simulink model "Impedance"  (R2020a)
settings: Solver=VariableStepAuto  StartTime=0.0  StopTime=2.0  RelTol=1e-3
values from neighbouring files (symbols this model uses):
  g = 9.81    [params.m]
  KD = 2*z*w    [params.m]
  KP = w^2    [params.m]
  Md = diag([2 2 2 2 2 2])    [params.m]
libraries: vrlib x1
settings Model: Creator=Sebastiano  LastModifiedBy=Sebastiano

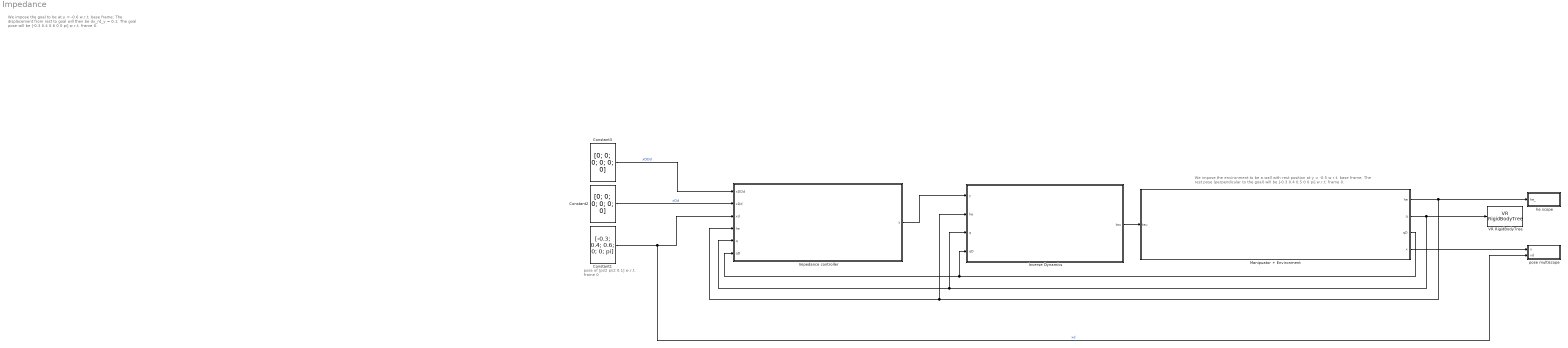
== system Impedance ==
  note: pose of [pi/2 pi/2 0.1]
      | w.r.t. frame 0
  note: We impose the environment to be a wall with rest position at y = -0.5 w.r.t. base frame;
      | The rest pose (perpendicular to the goal) will be [-0.3 0.4 0.5 0 0 pi] w.r.t. frame 0.
  note: We impose the goal to be at y = -0.6 w.r.t. base frame;
      | The displacement from rest to goal will then be dx_rd_y = 0.1;
      | The goal pose will be [-0.3 0.4 0.6 0 0 pi] w.r.t. frame 0.
  Constant1 : Constant  Value=[-0.3; 0.4; 0.6; 0; 0; pi]  VectorParams1D=off
  Constant2 : Constant  Value=[0; 0; 0; 0; 0; 0]  VectorParams1D=off
  Constant3 : Constant  Value=[0; 0; 0; 0; 0; 0]  VectorParams1D=off
  Impedance controller : Subsystem
  Inverse Dynamics : Subsystem
  Manipuator + Environment : Subsystem
  VR RigidBodyTree : vrlib/VR RigidBodyTree  RBT=robot  useRBT=on  Ts=-1  ForceViewerOpen=on
      settings: SourceProductBaseCode=SL
  he scope : Subsystem
  pose multiscope : Subsystem
  wires:
  Constant1/1 -> pose multiscope/2(xd), Impedance controller/3(xd)  "xd"
  Constant3/1 -> Impedance controller/1(xDDd)  "xDDd"
  Constant2/1 -> Impedance controller/2(xDd)  "xDd"
  Impedance controller/1(y) -> Inverse Dynamics/1(y)
  Manipuator + Environment/3(qD) -> Inverse Dynamics/4(qD), Impedance controller/6(qD)
  Manipuator + Environment/2(q) -> VR RigidBodyTree/1, Inverse Dynamics/3(q), Impedance controller/5(q)
  Inverse Dynamics/1(tau) -> Manipuator + Environment/1(tau)
  Manipuator + Environment/1(he) -> he scope/1(he_), Impedance controller/4(he), Inverse Dynamics/2(he)
  Manipuator + Environment/4(x) -> pose multiscope/1(x)

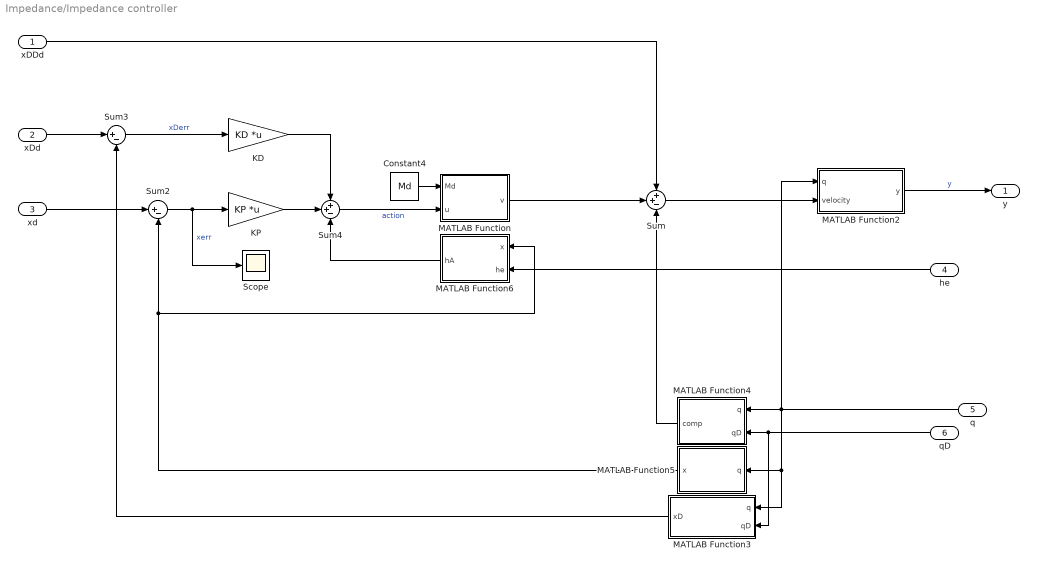
== system Impedance/Impedance controller ==
  xDDd : Inport
  xDd : Inport  Port=2
  xd : Inport  Port=3
  he : Inport  Port=4
  q : Inport  Port=5
  qD : Inport  Port=6
  Constant4 : Constant  Value=Md
  KD : Gain  Gain=KD  Multiplication=Matrix(K*u) (u vector)
  KP : Gain  Gain=KP  Multiplication=Matrix(K*u) (u vector)
  MATLAB Function : MATLAB Function  TreatAsAtomicUnit=on
  MATLAB Function2 : MATLAB Function  TreatAsAtomicUnit=on
  MATLAB Function3 : MATLAB Function  TreatAsAtomicUnit=on
  MATLAB Function4 : MATLAB Function  TreatAsAtomicUnit=on
  MATLAB Function5 : MATLAB Function  TreatAsAtomicUnit=on
  MATLAB Function6 : MATLAB Function  TreatAsAtomicUnit=on
  Scope : Scope
  Sum : Sum  Inputs=++-
  Sum2 : Sum  Inputs=|+-
  Sum3 : Sum  Inputs=|+-
  Sum4 : Sum  Inputs=++-
  y : Outport
  wires:
  Sum/1 -> MATLAB Function2/2(velocity)
  q/1 -> MATLAB Function3/1(q), MATLAB Function5/1(q), MATLAB Function4/1(q), MATLAB Function2/1(q)
  MATLAB Function5/1(x) -> Sum2/2, MATLAB Function6/1(x)
  xd/1 -> Sum2/1
  xDd/1 -> Sum3/1
  he/1 -> MATLAB Function6/2(he)
  Constant4/1 -> MATLAB Function/1(Md)
  MATLAB Function2/1(y) -> y/1  "y"
  qD/1 -> MATLAB Function4/2(qD), MATLAB Function3/2(qD)
  MATLAB Function3/1(xD) -> Sum3/2
  MATLAB Function4/1(comp) -> Sum/3
  Sum3/1 -> KD/1  "xDerr"
  xDDd/1 -> Sum/1
  KD/1 -> Sum4/1
  Sum2/1 -> Scope/1, KP/1  "xerr"
  KP/1 -> Sum4/2
  MATLAB Function/1(v) -> Sum/2
  Sum4/1 -> MATLAB Function/2(u)  "action"
  MATLAB Function6/1(hA) -> Sum4/3

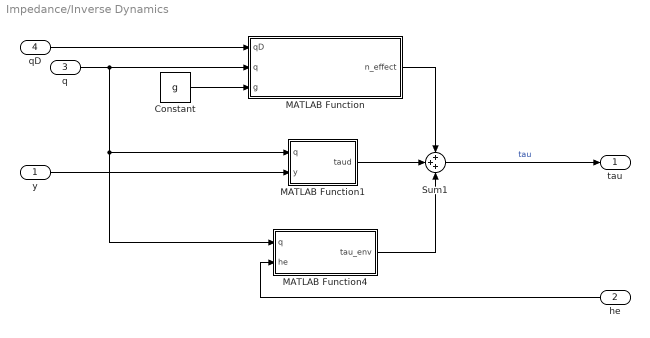
== system Impedance/Inverse Dynamics ==
  y : Inport
  he : Inport  Port=2
  q : Inport  Port=3
  qD : Inport  Port=4
  Constant : Constant  Value=g
  MATLAB Function : MATLAB Function  TreatAsAtomicUnit=on
  MATLAB Function1 : MATLAB Function  TreatAsAtomicUnit=on
  MATLAB Function4 : MATLAB Function  TreatAsAtomicUnit=on
  Sum1 : Sum  Inputs=+++
  tau : Outport
  wires:
  qD/1 -> MATLAB Function/1(qD)
  MATLAB Function/1(n_effect) -> Sum1/1
  MATLAB Function1/1(taud) -> Sum1/2
  q/1 -> MATLAB Function/2(q), MATLAB Function4/1(q), MATLAB Function1/1(q)
  Constant/1 -> MATLAB Function/3(g)
  y/1 -> MATLAB Function1/2(y)
  Sum1/1 -> tau/1  "tau"
  MATLAB Function4/1(tau_env) -> Sum1/3
  he/1 -> MATLAB Function4/2(he)

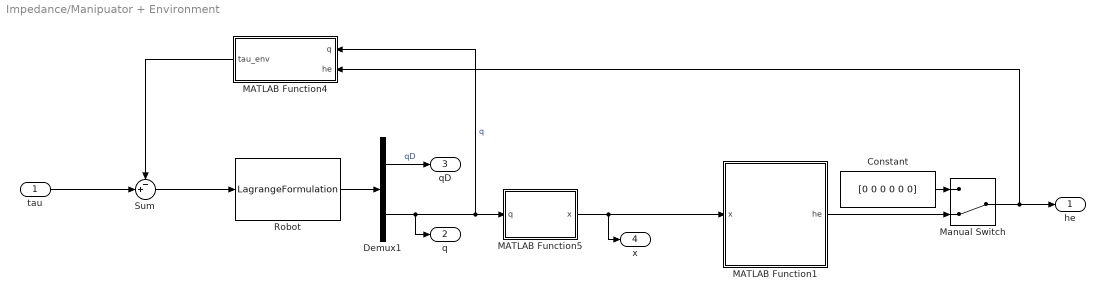
== system Impedance/Manipuator + Environment ==
  tau : Inport
  Constant : Constant  Value=[0 0 0 0 0 0]
  Demux1 : Demux  Outputs=[3, 3]
  MATLAB Function1 : MATLAB Function  TreatAsAtomicUnit=on
  MATLAB Function4 : MATLAB Function  TreatAsAtomicUnit=on
  MATLAB Function5 : MATLAB Function  TreatAsAtomicUnit=on
  Manual Switch : ManualSwitch  CurrentSetting=0
  Robot : S-Function  FunctionName=LagrangeFormulation  Parameters=g  SFunctionDeploymentMode=off  EnableBusSupport=off
  Sum : Sum  Inputs=-+|
  he : Outport
  q : Outport  Port=2
  qD : Outport  Port=3
  x : Outport  Port=4
  wires:
  Sum/1 -> Robot/1
  MATLAB Function1/1(he) -> Manual Switch/2
  Robot/1 -> Demux1/1
  MATLAB Function4/1(tau_env) -> Sum/1
  MATLAB Function5/1(x) -> x/1, MATLAB Function1/1(x)
  Constant/1 -> Manual Switch/1
  Manual Switch/1 -> MATLAB Function4/2(he), he/1
  Demux1/2 -> MATLAB Function4/1(q), MATLAB Function5/1(q), q/1  "q"
  tau/1 -> Sum/2
  Demux1/1 -> qD/1  "qD"

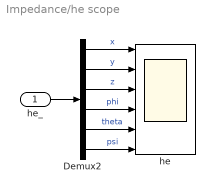
== system Impedance/he scope ==
  he_ : Inport
  Demux2 : Demux  Outputs=[1, 1, 1, 1, 1, 1]
  he : Scope  NumInputPorts=6
  wires:
  Demux2/4 -> he/4  "phi"
  Demux2/3 -> he/3  "z"
  Demux2/6 -> he/6  "psi"
  Demux2/5 -> he/5  "theta"
  Demux2/1 -> he/1  "x"
  he_/1 -> Demux2/1
  Demux2/2 -> he/2  "y"

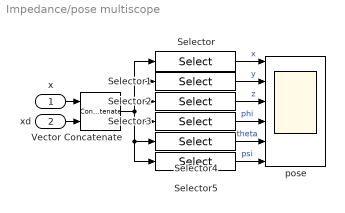
== system Impedance/pose multiscope ==
  x : Inport
  xd : Inport  Port=2
  Selector : Selector  NumberOfDimensions=2  InputPortWidth=3  IndexOptions=Index vector (dialog),Select all  Indices=1,7  OutputSizes=6,6
  Selector1 : Selector  NumberOfDimensions=2  InputPortWidth=3  IndexOptions=Index vector (dialog),Select all  Indices=2,7  OutputSizes=6,6
  Selector2 : Selector  NumberOfDimensions=2  InputPortWidth=3  IndexOptions=Index vector (dialog),Select all  Indices=3,7  OutputSizes=6,6
  Selector3 : Selector  NumberOfDimensions=2  InputPortWidth=3  IndexOptions=Index vector (dialog),Select all  Indices=4,7  OutputSizes=6,6
  Selector4 : Selector  NumberOfDimensions=2  InputPortWidth=3  IndexOptions=Index vector (dialog),Select all  Indices=5,7  OutputSizes=6,6
  Selector5 : Selector  NumberOfDimensions=2  InputPortWidth=3  IndexOptions=Index vector (dialog),Select all  Indices=6,7  OutputSizes=6,6
  Vector Concatenate : Concatenate  Mode=Multidimensional array  ConcatenateDimension=2
  pose : Scope  NumInputPorts=6
  wires:
  x/1 -> Vector Concatenate/1
  xd/1 -> Vector Concatenate/2
  Selector1/1 -> pose/2  "y"
  Selector5/1 -> pose/6  "psi"
  Selector3/1 -> pose/4  "phi"
  Selector/1 -> pose/1  "x"
  Selector4/1 -> pose/5  "theta"
  Vector Concatenate/1 -> Selector/1, Selector1/1, Selector2/1, Selector5/1, Selector4/1, Selector3/1
  Selector2/1 -> pose/3  "z"

== matlab function Impedance/Manipuator + Environment/MATLAB Function1 ==
  data: x input; he output
function he = environment(x)

% environment params
K = diag([2 2 2 0.1 0.1 0.1]);    % stiffness
wall = 0.5; % constraint position w.r.t. frame 0 (it's y=-0.5 w.r.t. base frame)

if x(3) >= wall  % check is done in frame 0
    % touching the environment! constrained motion
    % set up the rest position frame
    % (basically, same orientation as ee but position is the contact point at the wall)
    xr = x;
    xr(3) = wall;
    % calculate the forces
    dx_re = x - xr;
    he = K * dx_re;
else
    % free motion
    he = zeros(6,1);
end

he = reshape(he,[6 1]);

== matlab function Impedance/Manipuator + Environment/MATLAB Function4 ==
  data: q input; he input; tau_env output
function tau_env = J(q, he)

tau_env = Jacobian(q)' * he;

== matlab function Impedance/Impedance controller/MATLAB Function2 ==
  data: q input; y output; velocity input
function y = JAinv(q, velocity)

y = pinv(AnalyticalJacobian(q)) * velocity;

== matlab function Impedance/Impedance controller/MATLAB Function3 ==
  data: q input; xD output; qD input
function xD = JA(q, qD)

xD = AnalyticalJacobian(q)*qD;

== matlab function Impedance/Impedance controller/MATLAB Function4 ==
  data: q input; comp output; qD input
function comp = JAD(q, qD)

t1 = q(1);
t2 = q(2);
d3 = q(3);

Dt1 = qD(1);
Dt2 = qD(2);
Dd3 = qD(3);

JAD = [[ - 2/5*Dt1*cos(t1) - 3/10*cos(t1 + t2)*(Dt1 + Dt2), -3/10*cos(t1 + t2)*(Dt1 + Dt2), 0];
       [ - 3/10*sin(t1 + t2)*(Dt1 + Dt2) - 2/5*Dt1*sin(t1), -3/10*sin(t1 + t2)*(Dt1 + Dt2), 0];
       [                                                 0,                              0, 0];
       [                                                 0,                              0, 0];
       [                                                 0,                              0, 0];
       [                                                 0,                              0, 0]];

comp = JAD*qD;

== matlab function Impedance/Impedance controller/MATLAB Function5 ==
  data: q input; x output
function x = K(q)

t1 = q(1);
t2 = q(2);
d3 = q(3);

K = [[ cos(t1 + t2), -sin(t1 + t2), 0, (3*cos(t1 + t2))/10 + (2*cos(t1))/5]
     [ sin(t1 + t2),  cos(t1 + t2), 0, (3*sin(t1 + t2))/10 + (2*sin(t1))/5]
     [            0,             0, 1,                            d3 + 2/5]
     [            0,             0, 0,                                   1]];

pos = K(1:3, 4);
ori = rotm2eul(K(1:3,1:3), 'ZYZ')';

x = [pos; ori];

== matlab function Impedance/Inverse Dynamics/MATLAB Function ==
  data: qD input; q input; n_effect output; g input
function n_effect = n(qD, q, g)

n_effect = C_Lagrangian(q, qD)*qD + G_Lagrangian(q, g);

== matlab function Impedance/Inverse Dynamics/MATLAB Function1 ==
  data: q input; taud output; y input
function taud = B(q, y)

taud = B_Lagrangian(q)*y;

== matlab function Impedance/Impedance controller/MATLAB Function ==
  data: Md input; u input; v output
function v = Mdinv(Md, u)

v = Md \ u;

== matlab function Impedance/Impedance controller/MATLAB Function6 ==
  data: x input; hA output; he input
function hA = TAT(x,he)

ori = x(4:6);
hA = TransformAnalitical(ori)' * he;

== matlab function Impedance/Manipuator + Environment/MATLAB Function5 ==
  data: q input; x output
function x = K(q)

t1 = q(1);
t2 = q(2);
d3 = q(3);

K = [[ cos(t1 + t2), -sin(t1 + t2), 0, (3*cos(t1 + t2))/10 + (2*cos(t1))/5]
     [ sin(t1 + t2),  cos(t1 + t2), 0, (3*sin(t1 + t2))/10 + (2*sin(t1))/5]
     [            0,             0, 1,                            d3 + 2/5]
     [            0,             0, 0,                                   1]];

pos = K(1:3, 4);
ori = rotm2eul(K(1:3,1:3), 'ZYZ')';

x = [pos; ori];

== matlab function Impedance/Inverse Dynamics/MATLAB Function4 ==
  data: q input; he input; tau_env output
function tau_env = J(q, he)

tau_env = Jacobian(q)' * he;
